simulink model "sl_subsys_enab1"  (Simulink 7.6)
settings: Solver=FixedStepDiscrete  SolverMode=SingleTasking  StartTime=0.0  StopTime=25  FixedStep=.25  RelTol=1e-3
Description:
  | Comparison of enable port and outport settings
  | 
  | In the Reset subsystem, the state values are reset when the subsystem
  | is enabled and the output values are reset when the subsystem is disabled.
  | In the Held subsystem, the state and output values are held.
settings Model: Creator=The MathWorks Inc.  CovMetricSettings=d  ExtModeAutoUpdateStatusClock=off
settings OptimizationCC: BlockReduction=off  BooleanDataType=off  InitFltsAndDblsToZero=on
settings DebuggingCC: SaveWithParameterizedLinksMsg=none  SignalResolutionControl=TryResolveAllWithWarning  SolverPrmCheckMsg=none  MultiTaskDSMMsg=warning  MultiTaskCondExecSysMsg=none
settings HardwareCC: TargetUnknown=on
settings RTWCC: IncludeERTFirstTime=on
settings CodeAppCC: CustomSymbolStrFcn=$F$N$M
settings GRTTargetCC: TargetFcnLib=ansi_tfl_tmw.mat

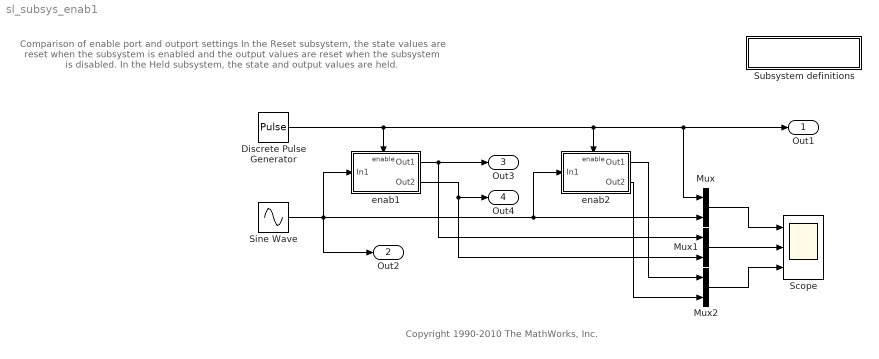
== system sl_subsys_enab1 ==
  note: Comparison of enable port and outport settings
      |
      | In the Reset subsystem, the state values are reset when the subsystem
      | is enabled and the output values are reset when the subsystem is disabled.
      | In the Held subsystem, the state and output values are held.
  note: Copyright 1990-2010 The MathWorks, Inc.
  " Subsystem definitions" : Subsystem
      settings: OpenFcn=helpview([matlabroot,'/toolbox/simulink/simdemos/simfeatures/html/sl_subsys_definitions.html']);
      mask Display: disp('Subsystem\ndefinitions')
  Discrete Pulse Generator : DiscretePulseGenerator  Period=20  PulseWidth=10  SampleTime=.25
  Mux : Mux  Inputs=2
  Mux1 : Mux  Inputs=2
  Mux2 : Mux  Inputs=2
  Scope : Scope  NumInputPorts=3
      settings: TimeRange=25  YMin=-5~-5~-5  YMax=5~5~5
  Sine Wave : Sin  SineType=Sample based  Amplitude=2  Samples=20  SampleTime=.25
  enab1 : Subsystem  TreatAsAtomicUnit=on
  enab2 : Subsystem  TreatAsAtomicUnit=on
  Out1 : Outport
  Out2 : Outport  Port=2
  Out3 : Outport  Port=3
  Out4 : Outport  Port=4
  wires:
  enab1/1(Out1) -> Out3/1, Mux1/1
  enab2/1(Out1) -> Mux2/1
  Discrete Pulse Generator/1 -> Out1/1, Mux/1, enab2/Enable, enab1/Enable
  Sine Wave/1 -> enab1/1(In1), enab2/1(In1), Mux/2, Out2/1
  Mux/1 -> Scope/1
  Mux1/1 -> Scope/2
  enab1/2(Out2) -> Out4/1, Mux1/2
  Mux2/1 -> Scope/3
  enab2/2(Out2) -> Mux2/2

== system sl_subsys_enab1/ Subsystem definitions ==

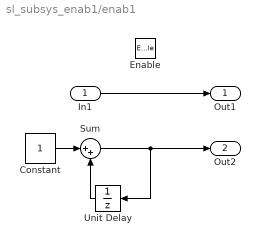
== system sl_subsys_enab1/enab1 ==
  In1 : Inport
  Enable : EnablePort  StatesWhenEnabling=reset
      settings: AttributesFormatString=States when enabling = %<StatesWhenEnabling>
  Constant : Constant
  Sum : Sum  Inputs=|++  SaturateOnIntegerOverflow=on  InputSameDT=on  OutDataTypeStr=Inherit: Same as first input
  Unit Delay : UnitDelay  SampleTime=.25
  Out1 : Outport  OutputWhenDisabled=reset  InitialOutput=5
      settings: AttributesFormatString=IC=%<InitialOutput>\nOutput when disabled=%<OutputWhenDisabled>
  Out2 : Outport  Port=2
      settings: AttributesFormatString=IC = %<InitialOutput>\nOutput when disabled = %<OutputWhenDisabled>
  wires:
  In1/1 -> Out1/1
  Sum/1 -> Out2/1, Unit Delay/1
  Constant/1 -> Sum/1
  Unit Delay/1 -> Sum/2

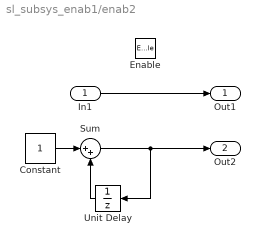
== system sl_subsys_enab1/enab2 ==
  In1 : Inport
  Enable : EnablePort
      settings: AttributesFormatString=States when enabling = %<StatesWhenEnabling>
  Constant : Constant
  Sum : Sum  Inputs=|++  SaturateOnIntegerOverflow=on  InputSameDT=on  OutDataTypeStr=Inherit: Same as first input
  Unit Delay : UnitDelay  SampleTime=.25
  Out1 : Outport  InitialOutput=1
      settings: AttributesFormatString=IC=%<InitialOutput>\nOutput when disabled=%<OutputWhenDisabled>
  Out2 : Outport  Port=2
      settings: AttributesFormatString=IC = %<InitialOutput>\nOutput when disabled = %<OutputWhenDisabled>
  wires:
  Unit Delay/1 -> Sum/2
  Constant/1 -> Sum/1
  Sum/1 -> Unit Delay/1, Out2/1
  In1/1 -> Out1/1
